simulink model "hsm_profile"  (R2018b)
settings: Solver=FixedStepDiscrete  StartTime=0.0  StopTime=10  FixedStep=0.001  RelTol=1e-3
undefined symbols (not defined in the file or in its folder): DiscIntNeverNeededParam, Ts
libraries: peGeneralControl x2, powerlib_meascontrol x1
settings Model: Creator=acer  LastModifiedBy=Kamran
settings DebuggingCC: LibraryContextMissingDiagnostic=none
settings SFSimCC: SimUseLocalCustomCode=off
settings RTWCC: RTWUseLocalCustomCode=off

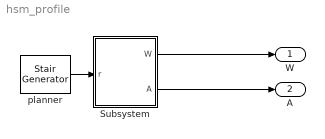
== system hsm_profile ==
  Subsystem : Subsystem
  planner : powerlib_meascontrol/Pulse & Signal Generators/Stair Generator  t=[0, 2, 5, 8]  e=[0, 1, 0.1, 0]  Ts=Ts
      settings: SourceProductName=Simscape Electrical
  W : Outport
  A : Outport  Port=2
  wires:
  Subsystem/1(W) -> W/1
  Subsystem/2(A) -> A/1
  planner/1 -> Subsystem/1(r)

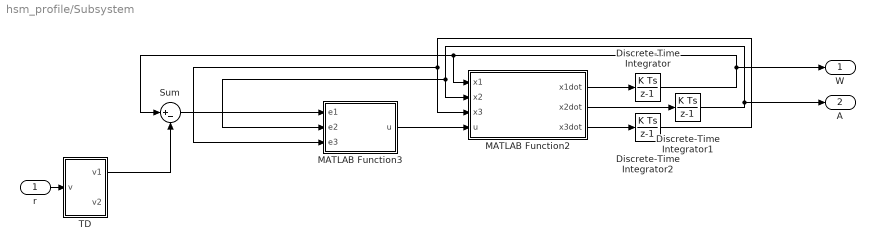
== system hsm_profile/Subsystem ==
  r : Inport
  Discrete-Time Integrator : DiscreteIntegrator  SampleTime=-1  ICPrevOutput=DiscIntNeverNeededParam  ICPrevScaledInput=DiscIntNeverNeededParam
  Discrete-Time Integrator1 : DiscreteIntegrator  SampleTime=-1  ICPrevOutput=DiscIntNeverNeededParam  ICPrevScaledInput=DiscIntNeverNeededParam
  Discrete-Time Integrator2 : DiscreteIntegrator  SampleTime=-1  ICPrevOutput=DiscIntNeverNeededParam  ICPrevScaledInput=DiscIntNeverNeededParam
  MATLAB Function2 : MATLAB Function  TreatAsAtomicUnit=on
  MATLAB Function3 : MATLAB Function  TreatAsAtomicUnit=on
  Sum : Sum  Inputs=|+-
  TD : Subsystem  mask{x3m=3, x2m=2, w=2 * pi * 120 / 60}
      mask prompts: x3m "x3 max"; x2m "x2 max"; w "w nominal"
  W : Outport
  A : Outport  Port=2
  wires:
  MATLAB Function2/3(x3dot) -> Discrete-Time Integrator2/1
  Discrete-Time Integrator2/1 -> MATLAB Function2/3(x3), MATLAB Function3/3(e3)
  MATLAB Function2/1(x1dot) -> Discrete-Time Integrator/1
  Discrete-Time Integrator/1 -> W/1, MATLAB Function2/1(x1), Sum/1
  MATLAB Function3/1(u) -> MATLAB Function2/4(u)
  Sum/1 -> MATLAB Function3/1(e1)
  MATLAB Function2/2(x2dot) -> Discrete-Time Integrator1/1
  TD/1(v1) -> Sum/2
  r/1 -> TD/1(v)
  Discrete-Time Integrator1/1 -> A/1, MATLAB Function3/2(e2), MATLAB Function2/2(x2)

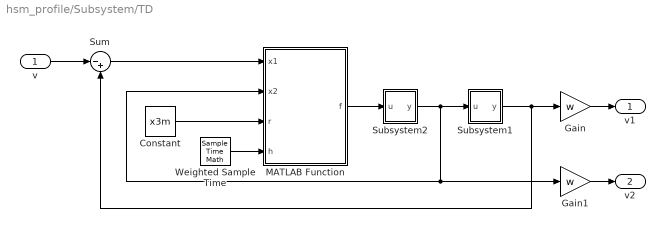
== system hsm_profile/Subsystem/TD ==
  v : Inport
  Constant : Constant  Value=x3m  SampleTime=-1
  Gain : Gain  Gain=w
  Gain1 : Gain  Gain=w
  MATLAB Function : MATLAB Function  TreatAsAtomicUnit=on
  Subsystem1 : Subsystem  mask{sat=inf, x0=0}
      mask Display: droots([], [0], 1);
  Subsystem2 : Subsystem  mask{sat=x2m, x0=0}
      mask Display: droots([], [0], 1);
  Sum : Sum  Inputs=|-+
  Weighted Sample Time : SampleTimeMath  TsampMathOp=Ts Only
  v1 : Outport
  v2 : Outport  Port=2
  wires:
  Subsystem2/1(y) -> Subsystem1/1(u), Gain1/1, MATLAB Function/2(x2)
  Subsystem1/1(y) -> Sum/2, Gain/1
  v/1 -> Sum/1
  Weighted Sample Time/1 -> MATLAB Function/4(h)
  Sum/1 -> MATLAB Function/1(x1)
  Constant/1 -> MATLAB Function/3(r)
  MATLAB Function/1(f) -> Subsystem2/1(u)
  Gain/1 -> v1/1
  Gain1/1 -> v2/1

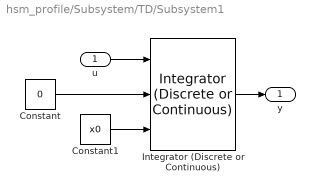
== system hsm_profile/Subsystem/TD/Subsystem1 ==
  u : Inport
  Constant : Constant  Value=0
  Constant1 : Constant  Value=x0
  Integrator (Discrete or Continuous) : peGeneralControl/Integrator (Discrete or Continuous)  LabelModeActiveChoice=Discrete  ExternalReset=level  LimitType=Anti-windup  B=sat  A=-sat  Ts=-1
  y : Outport
  wires:
  Constant1/1 -> Integrator (Discrete or Continuous)/3
  u/1 -> Integrator (Discrete or Continuous)/1
  Constant/1 -> Integrator (Discrete or Continuous)/2
  Integrator (Discrete or Continuous)/1 -> y/1

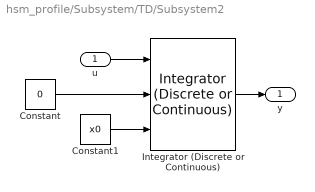
== system hsm_profile/Subsystem/TD/Subsystem2 ==
  u : Inport
  Constant : Constant  Value=0
  Constant1 : Constant  Value=x0
  Integrator (Discrete or Continuous) : peGeneralControl/Integrator (Discrete or Continuous)  LabelModeActiveChoice=Discrete  ExternalReset=level  LimitType=Anti-windup  B=sat  A=-sat  Ts=-1
  y : Outport
  wires:
  Integrator (Discrete or Continuous)/1 -> y/1
  Constant/1 -> Integrator (Discrete or Continuous)/2
  u/1 -> Integrator (Discrete or Continuous)/1
  Constant1/1 -> Integrator (Discrete or Continuous)/3

== matlab function hsm_profile/Subsystem/MATLAB Function2 ==
  data: x1 input; x2 input; x3 input; u input; x1dot output; x2dot output; x3dot output
function [x1dot,x2dot,x3dot] = fcn(x1,x2,x3,u)
x1dot=x2;
x2dot=x3;
x3dot=u;

== matlab function hsm_profile/Subsystem/MATLAB Function3 ==
  data: e1 input; u output; e2 input; e3 input
function u = fcn(e1,e2,e3)
a=10;    
b=a;
c=a;

u= -a*b*c*e1 -((a+b)*c + a*b)*e2 -(a+b+c)*e3;

% eta=100;
% landa=150;
% sigma=1;
% s=e3+2*landa*e2+landa^2*e1;
% u=-2*landa*e3 - landa^2*e2 - eta*tanh(s/sigma) + xddd;

== matlab function hsm_profile/Subsystem/TD/MATLAB Function ==
  data: x1 input; f output; x2 input; r input; h input
function f = fhan(x1, x2, r, h)

    d = r * h^2;
    a0 = h * x2;
    y = x1 + a0;
    a1 = sqrt(d * (d + 8 * abs(y)));
    a2 = a0 + sign(y) * (a1 - d) / 2;
    sy = (sign(y + d) - sign(y - d)) / 2;
    a = (a0 + y - a2) * sy + a2;
    sa = (sign(a + d) - sign(a - d)) / 2;
    f = -r * (a / d - sign(a)) * sa - r * sign(a);

end
